simulink model "Main"  (R2020a)
settings: Solver=VariableStepAuto  StartTime=0.0  StopTime=30  RelTol=1e-3
values from neighbouring files (symbols this model uses):
  A_eq = double(A_eq)    [source_export.m]
  B_eq = double(B_eq)    [source_export.m]
  C = [1 0 0 0 0 0 0 0 0 0 0 0 ... (first row only)    [source_export.m]
  C_simulink = eye(12)    [source_export.m]
  Condition_0 = transpose([0 0 0 0 0 0 0 0 0 0 0 0])    [source_export.m]
  Condition_1 = transpose([0.2 0.2 0.2 0.2 0.2 0.2 0.2 0.2 0.2 0.2 0.2 0.2])    [source_export.m]
  D = zeros(4,4)    [source_export.m]
  D_Simulink = zeros(12,4)    [source_export.m]
  g = 9.81    [source_export.m]
  inv_G0 = inv_G_0( : , [1 , 2 ,3 ,6])    [source_export.m]
  inv_G0_LQR = inv_G_0_LQR( : , [1 , 2 ,3 ,6])    [source_export.m]
  Ixx = 8.5532e-3    (= 0.0085532)    [source_export.m]
  Iyy = 8.5532e-3    (= 0.0085532)    [source_export.m]
  Izz = 1.476e-2    (= 0.01476)    [source_export.m]
  K_q_LQR = K_LQR(:,12+1:12+4)    [source_export.m]
  K_q_LQRk = K_LQRk(:,12+1:12+4)    [source_export.m]
  Kfeedback = place(A_eq,B_eq,Poles)    [source_export.m]
  m = 1    [source_export.m]
undefined symbols (not defined in the file or in its folder): K_LQR1
libraries: simulink x1
settings Model: Creator=ali14  LastModifiedBy=ali14
settings DebuggingCC: UnconnectedInputMsg=none  UnconnectedOutputMsg=none  UnconnectedLineMsg=none  SFMachineParentedDataDiag=error
settings ModelReferenceCC: EnableRefExpFcnMdlSchedulingChecks=off
settings RTWCC: Description=Generic Real-Time Target

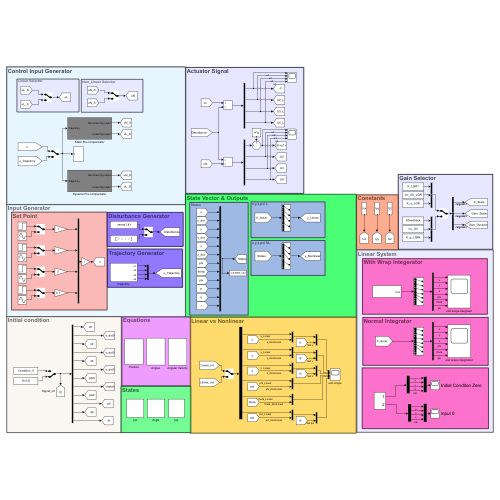
[thumbnail: Simulink's stored preview of the top-level diagram]
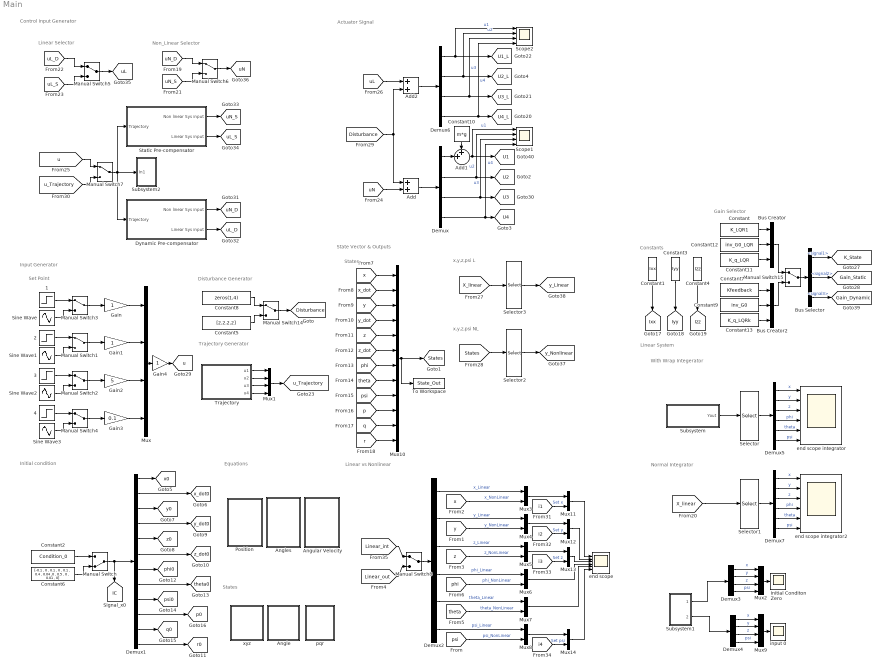
== system Main ==
  note: Gain Selector
  note: Actuator Signal
  note: States
  note: x,y,z,psi NL
  note: x,y,z,psi L
  note: Normal Integrator
  note: Trajectory Generator
  note: Linear Selector
  note: Non_Linear Selector
  note: Set Point
  note: Disturbance Generator
  note: State Vector & Outputs
  note: With Wrap Integerator
  note: Linear System
  note: Linear vs Nonlinear
  note: Constants
  note: Initial condition
  note: States
  note: Equations
  note: Input Generator
  note: Control Input Generator
  1 : Step  Time=3  SampleTime=0
  2 : Step  Time=3  SampleTime=0
  3 : Step  Time=0  SampleTime=0
  4 : Step  Time=5  SampleTime=0
  Add : Sum
  Add1 : Sum  Inputs=++|
  Add2 : Sum
  Angle : Subsystem
  Angles : Subsystem
  Angular Velocity : Subsystem
  Bus Creator : BusCreator  Inputs=3
  Bus Creator2 : BusCreator  Inputs=3
  Bus Selector : BusSelector  OutputSignals=signal1,signal2,signal3
  Constant : Constant  Value=K_LQR1
  Constant1 : Constant  Value=Ixx
  Constant10 : Constant  Value=m*g
  Constant11 : Constant  Value=K_q_LQR
  Constant12 : Constant  Value=inv_G0_LQR
  Constant13 : Constant  Value=K_q_LQRk
  Constant2 : Constant  Value=Condition_0
  Constant3 : Constant  Value=Iyy
  Constant4 : Constant  Value=Izz
  Constant5 : Constant  Value=[2,2,2,2]
  Constant6 : Constant  Value=[-0.1 , 0 , 0.1 , 0 , 0.1 , 0.4 , 0.04 ,0 , 0.5 , 0 , 0.01 , 0]
  Constant7 : Constant  Value=Kfeedback
  Constant8 : Constant  Value=zeros(1,4)
  Constant9 : Constant  Value=inv_G0
  Demux{,3..4,6} (4 alike) : Demux
  Demux1 : Demux  Outputs=12
  Demux2 : Demux  Outputs=6
  Demux5 : Demux  Outputs=6
  Demux7 : Demux  Outputs=6
  Dynamic Pre-compensator : Subsystem
  Gain : Gain
  Gain1 : Gain
  Gain2 : Gain  Gain=5
  Gain3 : Gain  Gain=0.1
  Gain4 : Gain
  Initial Conditon Zero : Scope
  Manual Switch : ManualSwitch  CurrentSetting=0
  Manual Switch{1..8,14..15} (10 alike) : ManualSwitch
  Mux{,1..2,9} (4 alike) : Mux
  Mux10 : Mux  Inputs=12
  Mux{3..8,11..14} (10 alike) : Mux  Inputs=2
  Position : Subsystem
  Scope1 : Scope  NumInputPorts=4
  Scope2 : Scope  NumInputPorts=4
  Selector : Selector  InputPortWidth=12  IndexOptions=Index vector (dialog)  Indices=[1 3 5 7 8 9]  OutputSizes=1
  Selector1 : Selector  InputPortWidth=12  IndexOptions=Index vector (dialog)  Indices=[1 3 5 7 8 9]  OutputSizes=1
  Selector2 : Selector  InputPortWidth=12  IndexOptions=Index vector (dialog)  Indices=[1 3 5 9]  OutputSizes=1
  Selector3 : Selector  InputPortWidth=12  IndexOptions=Index vector (dialog)  Indices=[1 3 5 9]  OutputSizes=1
  Sine Wave{,1..3} (4 alike) : Sin  SampleTime=0
  Static Pre-compensator : Subsystem
  Subsystem : Subsystem
  Subsystem1 : Subsystem
  Subsystem2 : Subsystem
  To Workspace : ToWorkspace  VariableName=State_Out  SampleTime=-1
  "Trajectory " : Subsystem
  end scope : Scope  NumInputPorts=6
  end scope integrator : Scope  NumInputPorts=6
  end scope integrator2 : Scope  NumInputPorts=6
  input 0 : Scope
  pqr : Subsystem
  xyz : Subsystem
  tag scope: Disturbance=global, Gain_Dynamic=global, Gain_Static=global, IC=global, Ixx=global, Iyy=global, Izz=global, K_State=global, States=global, U1=global, U1_L=global, U2=global, U2_L=global, U3=global, U3_L=global, U4=global, U4_L=global, p0=global, phi0=global, psi0=global, q0=global, r0=global, theta0=global, u=global, uL=global, uL_D=global, uL_S=global, uN=global, uN_D=global, uN_S=global, u_Trajectory=global, x0=global, x_dot0=global, y0=global, y_Linear=global, y_Nonlinear=global, y_dot0=global, z0=global, z_dot0=global
  wires:
  Demux1/1 -> [x0]
  Demux1/3 -> [y0]
  Demux1/5 -> [z0]
  Demux1/2 -> [x_dot0]
  Demux1/4 -> [y_dot0]
  Demux1/6 -> [z_dot0]
  Demux1/7 -> [phi0]
  Demux1/8 -> [theta0]
  Demux1/9 -> [psi0]
  Demux1/10 -> [p0]
  Demux1/11 -> [q0]
  Demux1/12 -> [r0]
  Constant1/1 -> [Ixx]
  Constant3/1 -> [Iyy]
  Constant4/1 -> [Izz]
  Constant6/1 -> Manual Switch/2
  Manual Switch/1 -> Demux1/1, [IC]
  Constant2/1 -> Manual Switch/1
  Demux2/1 -> Mux3/1  "x_Linear"
  [x] -> Mux3/2  "x_NonLinear"
  Demux2/2 -> Mux4/1  "y_Linear"
  Demux2/3 -> Mux5/1  "z_Linear"
  Demux2/4 -> Mux6/1  "phi_Linear"
  Demux2/5 -> Mux7/1  "theta_Linear"
  Demux2/6 -> Mux8/1  "psi_Linear"
  [y] -> Mux4/2  "y_NonLinear"
  [z] -> Mux5/2  "z_NonLinear"
  [phi] -> Mux6/2  "phi_NonLinear"
  [psi] -> Mux8/2  "psi_NonLinear"
  [theta] -> Mux7/2  "theta_NonLinear"
  Mux6/1 -> end scope/4
  Mux7/1 -> end scope/5
  Subsystem1/1(Outport) -> Demux3/1
  Demux3/1 -> Mux2/1  "x"
  Demux3/2 -> Mux2/2  "y"
  Demux3/3 -> Mux2/3  "z"
  Demux3/4 -> Mux2/4  "psi"
  Mux2/1 -> Initial Conditon Zero/1
  Demux4/2 -> Mux9/2  "y"
  Demux4/1 -> Mux9/1  "x"
  Demux4/4 -> Mux9/4  "psi"
  Demux4/3 -> Mux9/3  "z"
  Subsystem1/2(Outport1) -> Demux4/1
  Mux9/1 -> input 0/1
  Subsystem/1(Yout) -> Selector/1
  Selector/1 -> Demux5/1
  Demux5/1 -> end scope integrator/1  "x"
  Demux5/2 -> end scope integrator/2  "y"
  Demux5/3 -> end scope integrator/3  "z"
  Demux5/4 -> end scope integrator/4  "phi"
  Demux5/5 -> end scope integrator/5  "theta"
  Demux5/6 -> end scope integrator/6  "psi"
  [x] -> Mux10/1
  [x_dot] -> Mux10/2
  [y] -> Mux10/3
  [y_dot] -> Mux10/4
  [z] -> Mux10/5
  [z_dot] -> Mux10/6
  [phi] -> Mux10/7
  [theta] -> Mux10/8
  [psi] -> Mux10/9
  [p] -> Mux10/10
  [q] -> Mux10/11
  [r] -> Mux10/12
  3/1 -> Manual Switch2/1
  Gain2/1 -> Mux/3
  1/1 -> Manual Switch3/1
  Manual Switch4/1 -> Gain3/1
  Manual Switch2/1 -> Gain2/1
  Sine Wave2/1 -> Manual Switch2/2
  Gain3/1 -> Mux/4
  4/1 -> Manual Switch4/1
  Sine Wave3/1 -> Manual Switch4/2
  Sine Wave/1 -> Manual Switch3/2
  Gain/1 -> Mux/1
  Gain1/1 -> Mux/2
  Sine Wave1/1 -> Manual Switch1/2
  2/1 -> Manual Switch1/1
  Manual Switch1/1 -> Gain1/1
  Demux7/2 -> end scope integrator2/2  "y"
  Demux7/6 -> end scope integrator2/6  "psi"
  Demux7/4 -> end scope integrator2/4  "phi"
  [X_linear] -> Selector1/1
  Demux7/3 -> end scope integrator2/3  "z"
  Demux7/5 -> end scope integrator2/5  "theta"
  Selector1/1 -> Demux7/1
  Demux7/1 -> end scope integrator2/1  "x"
  Manual Switch14/1 -> [Disturbance]
  Constant8/1 -> Manual Switch14/1
  Constant5/1 -> Manual Switch14/2
  Bus Selector/1 -> [K_State]  "<signal1>"
  Demux6/1 -> Scope2/1, [U1_L]  "u1"
  Demux6/3 -> Scope2/3, [U3_L]  "u3"
  Demux6/2 -> Scope2/2, [U2_L]  "u2"
  Demux6/4 -> Scope2/4, [U4_L]  "u4"
  Demux/1 -> Add1/2
  Demux/4 -> Scope1/4, [U4]  "u4"
  Demux/3 -> Scope1/3, [U3]  "u3"
  Constant10/1 -> Add1/1
  Demux/2 -> Scope1/2, [U2]  "u2"
  Add1/1 -> Scope1/1, [U1]  "u1"
  Static Pre-compensator/2(Linear Sys input) -> [uL_S]
  Static Pre-compensator/1(Non linear Sys input) -> [uN_S]
  Dynamic Pre-compensator/2(Linear Sys input) -> [uL_D]
  Dynamic Pre-compensator/1(Non linear Sys input) -> [uN_D]
  [uN_D] -> Manual Switch6/1
  [uN_S] -> Manual Switch6/2
  [uL_S] -> Manual Switch5/2
  [uL_D] -> Manual Switch5/1
  Manual Switch6/1 -> [uN]
  Manual Switch5/1 -> [uL]
  Selector3/1 -> [y_Linear]
  Selector2/1 -> [y_Nonlinear]
  [X_linear] -> Selector3/1
  Mux10/1 -> [States], To Workspace/1
  [States] -> Selector2/1
  [uN] -> Add/2
  [Disturbance] -> Add2/2, Add/1
  Add2/1 -> Demux6/1
  Add/1 -> Demux/1
  [uL] -> Add2/1
  Constant/1 -> Bus Creator/1
  Constant12/1 -> Bus Creator/2
  Constant7/1 -> Bus Creator2/1
  Constant9/1 -> Bus Creator2/2
  Bus Creator/1 -> Manual Switch15/1
  Bus Creator2/1 -> Manual Switch15/2
  Manual Switch15/1 -> Bus Selector/1
  Bus Selector/2 -> [Gain_Static]  "<signal2>"
  Constant11/1 -> Bus Creator/3
  Constant13/1 -> Bus Creator2/3
  Bus Selector/3 -> [Gain_Dynamic]  "<signal3>"
  [u_Trajectory] -> Manual Switch7/2
  [u] -> Manual Switch7/1
  Manual Switch7/1 -> Dynamic Pre-compensator/1(Trajectory), Subsystem2/1(In1), Static Pre-compensator/1(Trajectory)
  "Trajectory "/4(u4) -> Mux1/4
  Mux1/1 -> [u_Trajectory]
  "Trajectory "/1(u1) -> Mux1/1
  "Trajectory "/2(u2) -> Mux1/2
  "Trajectory "/3(u3) -> Mux1/3
  Mux3/1 -> Mux11/1
  [i1] -> Mux11/2  "Set x"
  Mux11/1 -> end scope/1
  [i2] -> Mux12/2  "Set y"
  Mux4/1 -> Mux12/1
  Mux12/1 -> end scope/2
  [i3] -> Mux13/2  "Set z"
  Mux5/1 -> Mux13/1
  Mux13/1 -> end scope/3
  [i4] -> Mux14/2  "Set psi"
  Mux8/1 -> Mux14/1
  Mux14/1 -> end scope/6
  Manual Switch8/1 -> Demux2/1
  [Linear_out] -> Manual Switch8/2
  [Linear_int] -> Manual Switch8/1
  Manual Switch3/1 -> Gain/1
  Mux/1 -> Gain4/1
  Gain4/1 -> [u]

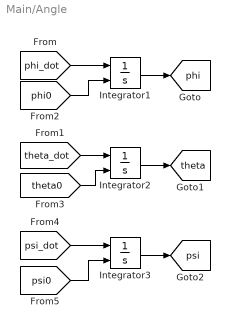
== system Main/Angle ==
  Integrator1 : Integrator  InitialConditionSource=external  WrapState=on
  Integrator2 : Integrator  InitialConditionSource=external  WrapState=on
  Integrator3 : Integrator  InitialConditionSource=external  WrapState=on
  tag scope: phi=global, psi=global, theta=global
  wires:
  Integrator2/1 -> [theta]
  [theta_dot] -> Integrator2/1
  Integrator3/1 -> [psi]
  [theta0] -> Integrator2/2
  [psi_dot] -> Integrator3/1
  [phi0] -> Integrator1/2
  Integrator1/1 -> [phi]
  [psi0] -> Integrator3/2
  [phi_dot] -> Integrator1/1

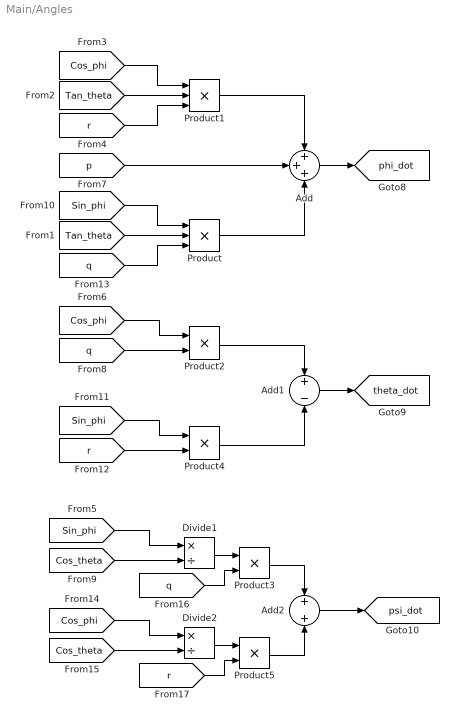
== system Main/Angles ==
  Add : Sum  Inputs=+++
  Add1 : Sum  Inputs=+-
  Add2 : Sum
  Divide1 : Product  Inputs=*/
  Divide2 : Product  Inputs=*/
  Product : Product  Inputs=3
  Product1 : Product  Inputs=3
  Product{2..5} (4 alike) : Product
  tag scope: phi_dot=global, psi_dot=global, theta_dot=global
  wires:
  [Sin_phi] -> Product/1
  [Tan_theta] -> Product/2
  [q] -> Product/3
  Product/1 -> Add/3
  [p] -> Add/2
  [Cos_phi] -> Product1/1
  [Tan_theta] -> Product1/2
  [r] -> Product1/3
  Product1/1 -> Add/1
  Add/1 -> [phi_dot]
  Add1/1 -> [theta_dot]
  [Cos_phi] -> Product2/1
  [q] -> Product2/2
  Product2/1 -> Add1/1
  Product4/1 -> Add1/2
  [Sin_phi] -> Divide1/1
  [Cos_theta] -> Divide1/2
  Divide1/1 -> Product3/1
  [r] -> Product4/2
  [Sin_phi] -> Product4/1
  Add2/1 -> [psi_dot]
  Product3/1 -> Add2/1
  [Cos_phi] -> Divide2/1
  Divide2/1 -> Product5/1
  [Cos_theta] -> Divide2/2
  Product5/1 -> Add2/2
  [q] -> Product3/2
  [r] -> Product5/2

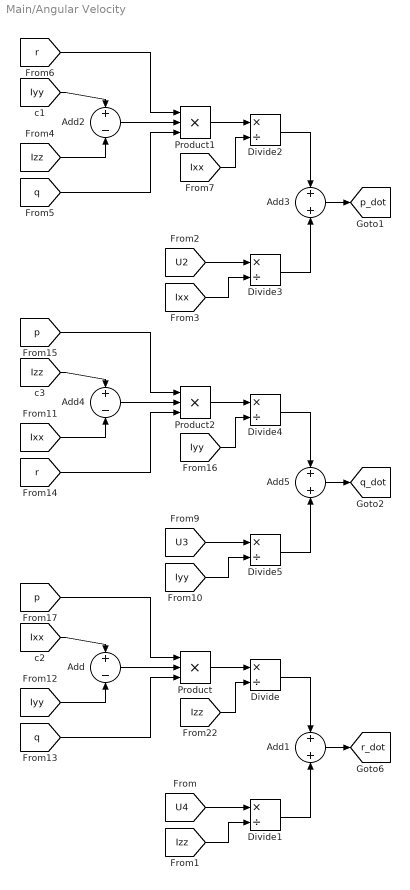
== system Main/Angular Velocity ==
  Add : Sum  Inputs=+-
  Add1 : Sum
  Add2 : Sum  Inputs=+-
  Add3 : Sum
  Add4 : Sum  Inputs=+-
  Add5 : Sum
  Divide{,1..5} (6 alike) : Product  Inputs=*/
  Product : Product  Inputs=3
  Product1 : Product  Inputs=3
  Product2 : Product  Inputs=3
  tag scope: p_dot=global, q_dot=global, r_dot=global
  wires:
  [Ixx] -> Add/1
  [Iyy] -> Add/2
  Add/1 -> Product/2
  [p] -> Product/1
  [q] -> Product/3
  Product/1 -> Divide/1
  [Izz] -> Divide/2
  Divide/1 -> Add1/1
  Add1/1 -> [r_dot]
  [U4] -> Divide1/1
  [Izz] -> Divide1/2
  Divide1/1 -> Add1/2
  [Izz] -> Add2/2
  Add2/1 -> Product1/2
  [r] -> Product1/1
  [U2] -> Divide3/1
  Add3/1 -> [p_dot]
  Divide2/1 -> Add3/1
  [Ixx] -> Divide3/2
  [q] -> Product1/3
  [Ixx] -> Divide2/2
  Product1/1 -> Divide2/1
  [Iyy] -> Add2/1
  Divide3/1 -> Add3/2
  [U3] -> Divide5/1
  [Iyy] -> Divide4/2
  Add5/1 -> [q_dot]
  [Iyy] -> Divide5/2
  Product2/1 -> Divide4/1
  [p] -> Product2/1
  Divide4/1 -> Add5/1
  [r] -> Product2/3
  Divide5/1 -> Add5/2
  [Ixx] -> Add4/2
  [Izz] -> Add4/1
  Add4/1 -> Product2/2

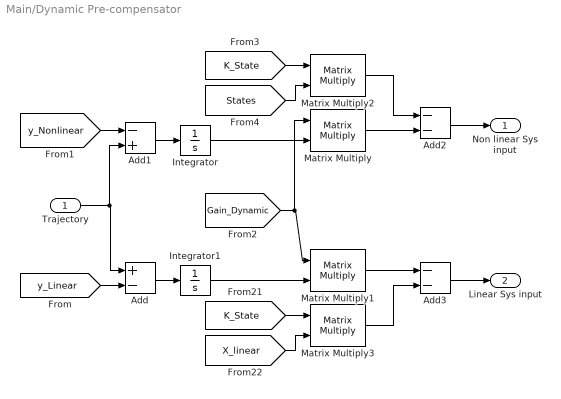
== system Main/Dynamic Pre-compensator ==
  Trajectory : Inport
  Add : Sum  Inputs=+-
  Add1 : Sum  Inputs=-+
  Add2 : Sum  Inputs=--
  Add3 : Sum  Inputs=--
  Integrator : Integrator
  Integrator1 : Integrator
  Matrix Multiply{,1..3} (4 alike) : Product  Multiplication=Matrix(*)
  Non linear Sys input : Outport
  Linear Sys input : Outport  Port=2
  wires:
  Trajectory/1 -> Add1/2, Add/1
  [y_Linear] -> Add/2
  [y_Nonlinear] -> Add1/1
  Add1/1 -> Integrator/1
  Add/1 -> Integrator1/1
  Integrator1/1 -> Matrix Multiply1/2
  [Gain_Dynamic] -> Matrix Multiply/1, Matrix Multiply1/1
  [K_State] -> Matrix Multiply3/1
  [States] -> Matrix Multiply2/2
  [K_State] -> Matrix Multiply2/1
  [X_linear] -> Matrix Multiply3/2
  Matrix Multiply/1 -> Add2/2
  Matrix Multiply2/1 -> Add2/1
  Matrix Multiply1/1 -> Add3/1
  Matrix Multiply3/1 -> Add3/2
  Add2/1 -> Non linear Sys input/1
  Add3/1 -> Linear Sys input/1
  Integrator/1 -> Matrix Multiply/2

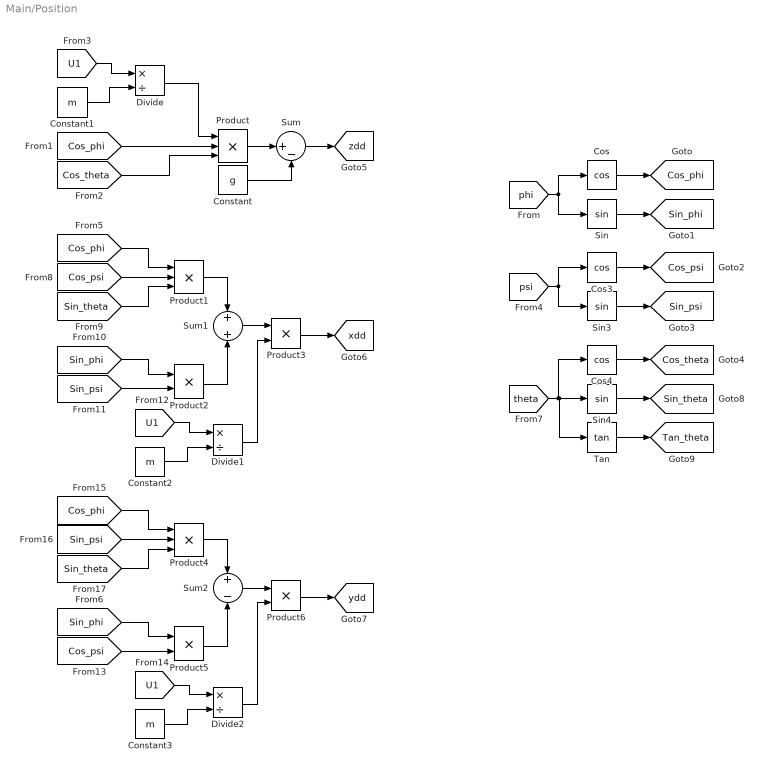
== system Main/Position ==
  Constant : Constant  Value=g
  Constant1 : Constant  Value=m
  Constant2 : Constant  Value=m
  Constant3 : Constant  Value=m
  Cos : Trigonometry  Operator=cos
  Cos3 : Trigonometry  Operator=cos
  Cos4 : Trigonometry  Operator=cos
  Divide : Product  Inputs=*/
  Divide1 : Product  Inputs=*/
  Divide2 : Product  Inputs=*/
  Product : Product  Inputs=3
  Product1 : Product  Inputs=3
  Product{2..3,5..6} (4 alike) : Product
  Product4 : Product  Inputs=3
  Sin : Trigonometry
  Sin3 : Trigonometry
  Sin4 : Trigonometry
  Sum : Sum  Inputs=|+-
  Sum1 : Sum
  Sum2 : Sum  Inputs=+-
  Tan : Trigonometry  Operator=tan
  tag scope: Cos_phi=global, Cos_psi=global, Cos_theta=global, Sin_phi=global, Sin_psi=global, Sin_theta=global, Tan_theta=global, xdd=global, ydd=global, zdd=global
  wires:
  Constant/1 -> Sum/2
  Product/1 -> Sum/1
  Sum/1 -> [zdd]
  Constant1/1 -> Divide/2
  [U1] -> Divide/1
  Divide/1 -> Product/1
  [phi] -> Cos/1, Sin/1
  Cos/1 -> [Cos_phi]
  Sin/1 -> [Sin_phi]
  Sin3/1 -> [Sin_psi]
  Cos3/1 -> [Cos_psi]
  [psi] -> Cos3/1, Sin3/1
  Sin4/1 -> [Sin_theta]
  Cos4/1 -> [Cos_theta]
  [theta] -> Cos4/1, Tan/1, Sin4/1
  [Cos_phi] -> Product/2
  [Cos_theta] -> Product/3
  [Cos_phi] -> Product1/1
  [Cos_psi] -> Product1/2
  [Sin_theta] -> Product1/3
  [Sin_psi] -> Product2/2
  [Sin_phi] -> Product2/1
  Product2/1 -> Sum1/2
  Product1/1 -> Sum1/1
  Product3/1 -> [xdd]
  Sum1/1 -> Product3/1
  Constant2/1 -> Divide1/2
  [U1] -> Divide1/1
  Divide1/1 -> Product3/2
  Product4/1 -> Sum2/1
  [Sin_theta] -> Product4/3
  Constant3/1 -> Divide2/2
  [Sin_psi] -> Product4/2
  [Cos_phi] -> Product4/1
  Product5/1 -> Sum2/2
  Divide2/1 -> Product6/2
  Sum2/1 -> Product6/1
  [Sin_phi] -> Product5/1
  [U1] -> Divide2/1
  [Cos_psi] -> Product5/2
  Product6/1 -> [ydd]
  Tan/1 -> [Tan_theta]

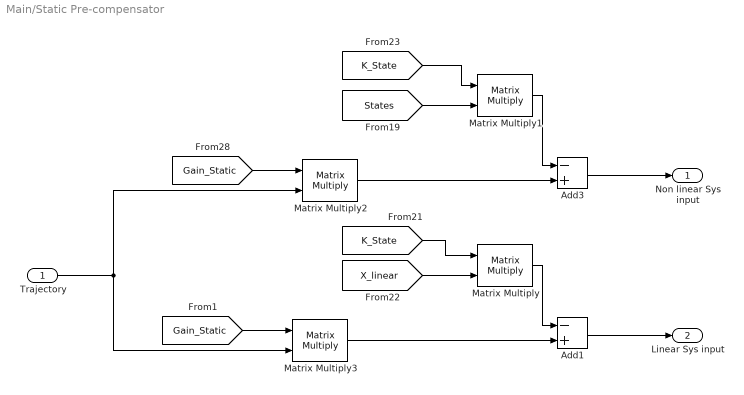
== system Main/Static Pre-compensator ==
  Trajectory : Inport
  Add1 : Sum  Inputs=-+
  Add3 : Sum  Inputs=-+
  Matrix Multiply{,1..3} (4 alike) : Product  Multiplication=Matrix(*)
  Non linear Sys input : Outport
  Linear Sys input : Outport  Port=2
  wires:
  Matrix Multiply1/1 -> Add3/1
  [States] -> Matrix Multiply1/2
  [K_State] -> Matrix Multiply1/1
  Add3/1 -> Non linear Sys input/1
  Matrix Multiply2/1 -> Add3/2
  [Gain_Static] -> Matrix Multiply2/1
  Matrix Multiply/1 -> Add1/1
  [X_linear] -> Matrix Multiply/2
  [K_State] -> Matrix Multiply/1
  Trajectory/1 -> Matrix Multiply3/2, Matrix Multiply2/2
  Matrix Multiply3/1 -> Add1/2
  [Gain_Static] -> Matrix Multiply3/1
  Add1/1 -> Linear Sys input/1

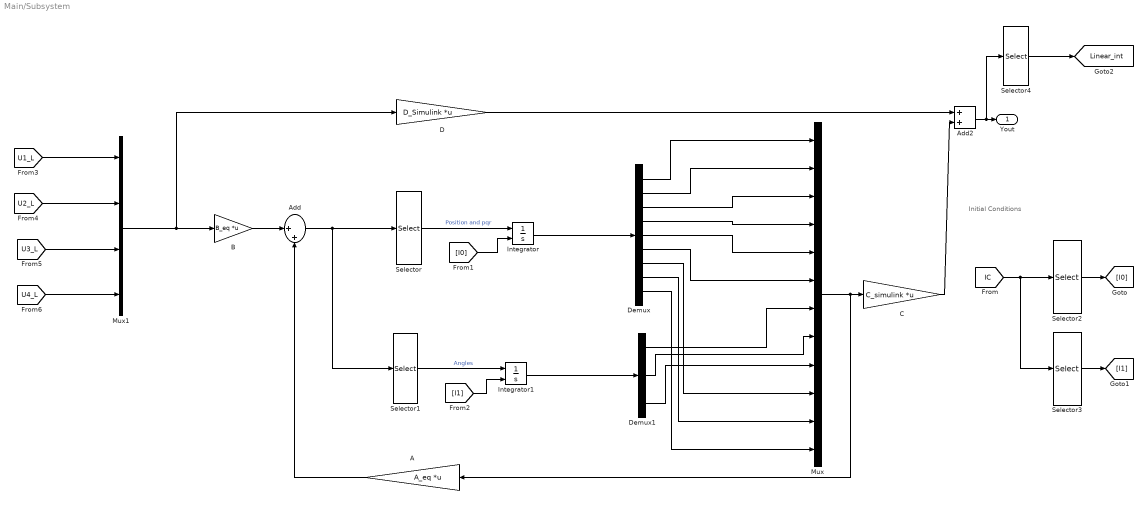
== system Main/Subsystem ==
  note: Initial Conditions
  A : Gain  Gain=A_eq  Multiplication=Matrix(K*u)
  Add : Sum  Inputs=|++
  Add2 : Sum
  B : Gain  Gain=B_eq  Multiplication=Matrix(K*u)
  C : Gain  Gain=C_simulink  Multiplication=Matrix(K*u)
  D : Gain  Gain=D_Simulink  Multiplication=Matrix(K*u)
  Demux : Demux  Outputs=9
  Demux1 : Demux  Outputs=3
  Integrator : Integrator  InitialConditionSource=external
  Integrator1 : Integrator  InitialConditionSource=external  WrapState=on
  Mux : Mux  Inputs=12
  Mux1 : Mux
  Selector : Selector  InputPortWidth=12  IndexOptions=Index vector (dialog)  Indices=[1 2 3 4 5 6 10 11 12]  OutputSizes=1
  Selector1 : Selector  InputPortWidth=12  IndexOptions=Index vector (dialog)  Indices=[7 8 9]  OutputSizes=1
  Selector2 : Selector  InputPortWidth=12  IndexOptions=Index vector (dialog)  Indices=[1 2 3 4 5 6 10 11 12]  OutputSizes=1
  Selector3 : Selector  InputPortWidth=12  IndexOptions=Index vector (dialog)  Indices=[7 8 9]  OutputSizes=1
  Selector4 : Selector  InputPortWidth=12  IndexOptions=Index vector (dialog)  Indices=[1 3 5 7 8 9]  OutputSizes=1
  Yout : Outport
  tag scope: Linear_int=global
  wires:
  B/1 -> Add/1
  A/1 -> Add/2
  Add/1 -> Selector1/1, Selector/1
  Selector/1 -> Integrator/1  "Position and pqr"
  Selector1/1 -> Integrator1/1  "Angles"
  [IC] -> Selector3/1, Selector2/1
  Selector3/1 -> [I1]
  Selector2/1 -> [I0]
  [I1] -> Integrator1/2
  [I0] -> Integrator/2
  Integrator1/1 -> Demux1/1
  Integrator/1 -> Demux/1
  Demux/1 -> Mux/1
  Demux/2 -> Mux/2
  Demux/3 -> Mux/3
  Demux/4 -> Mux/4
  Demux/5 -> Mux/5
  Demux/6 -> Mux/6
  Demux1/1 -> Mux/7
  Demux1/2 -> Mux/8
  Demux1/3 -> Mux/9
  Demux/7 -> Mux/10
  Demux/8 -> Mux/11
  Demux/9 -> Mux/12
  D/1 -> Add2/1
  C/1 -> Add2/2
  Mux1/1 -> D/1, B/1
  [U2_L] -> Mux1/2
  [U3_L] -> Mux1/3
  [U4_L] -> Mux1/4
  Add2/1 -> Selector4/1, Yout/1
  Mux/1 -> A/1, C/1
  [U1_L] -> Mux1/1
  Selector4/1 -> [Linear_int]

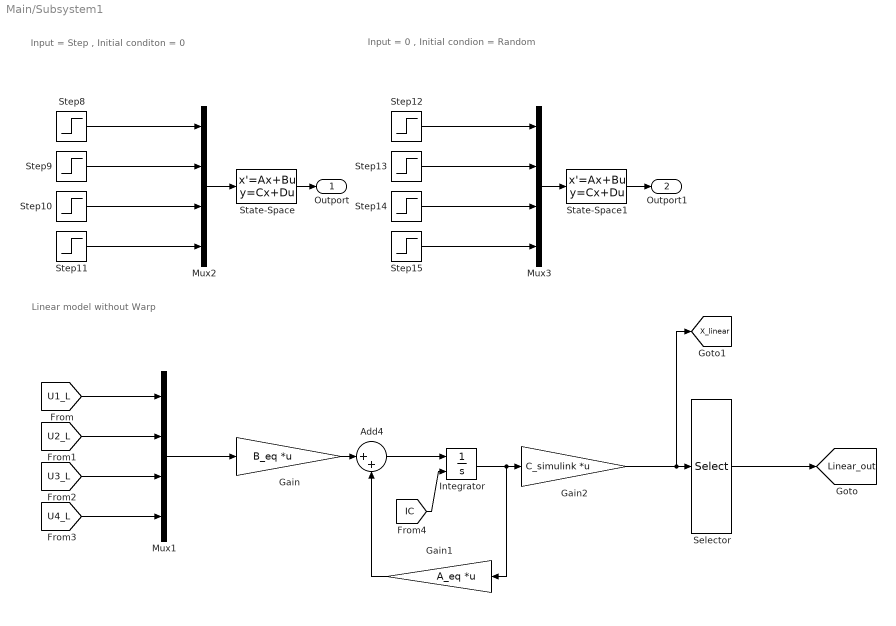
== system Main/Subsystem1 ==
  note: Linear model without Warp
  note: Input = Step , Initial conditon = 0
  note: Input = 0 , Initial condion = Random
  Add4 : Sum  Inputs=|++
  Gain : Gain  Gain=B_eq  Multiplication=Matrix(K*u)
  Gain1 : Gain  Gain=A_eq  Multiplication=Matrix(K*u)
  Gain2 : Gain  Gain=C_simulink  Multiplication=Matrix(K*u)
  Integrator : Integrator  InitialConditionSource=external
  Mux1 : Mux
  Mux2 : Mux
  Mux3 : Mux
  Selector : Selector  InputPortWidth=12  IndexOptions=Index vector (dialog)  Indices=[1 3 5 7 8 9]  OutputSizes=1
  State-Space : StateSpace  A=A_eq  B=B_eq  C=C  D=D  InitialCondition=Condition_0
  State-Space1 : StateSpace  A=A_eq  B=B_eq  C=C  D=D  InitialCondition=Condition_1
  Step{8..11} (4 alike) : Step  Time=0  SampleTime=0
  Step{12..15} (4 alike) : Step  Time=0  After=0  SampleTime=0
  Outport : Outport
  Outport1 : Outport  Port=2
  tag scope: Linear_out=global, X_linear=global
  wires:
  State-Space1/1 -> Outport1/1
  Step15/1 -> Mux3/4
  Step11/1 -> Mux2/4
  Step9/1 -> Mux2/2
  Mux3/1 -> State-Space1/1
  Step10/1 -> Mux2/3
  State-Space/1 -> Outport/1
  Step13/1 -> Mux3/2
  Mux2/1 -> State-Space/1
  Step14/1 -> Mux3/3
  [U2_L] -> Mux1/2
  [U3_L] -> Mux1/3
  [U4_L] -> Mux1/4
  Step12/1 -> Mux3/1
  [U1_L] -> Mux1/1
  Selector/1 -> [Linear_out]
  [IC] -> Integrator/2
  Integrator/1 -> Gain1/1, Gain2/1
  Gain1/1 -> Add4/2
  Mux1/1 -> Gain/1
  Gain/1 -> Add4/1
  Gain2/1 -> [X_linear], Selector/1
  Add4/1 -> Integrator/1
  Step8/1 -> Mux2/1

== system Main/Subsystem2 ==
  In1 : Inport
  Demux8 : Demux
  tag scope: i1=global, i2=global, i3=global, i4=global
  wires:
  In1/1 -> Demux8/1
  Demux8/1 -> [i1]
  Demux8/2 -> [i2]
  Demux8/3 -> [i3]
  Demux8/4 -> [i4]

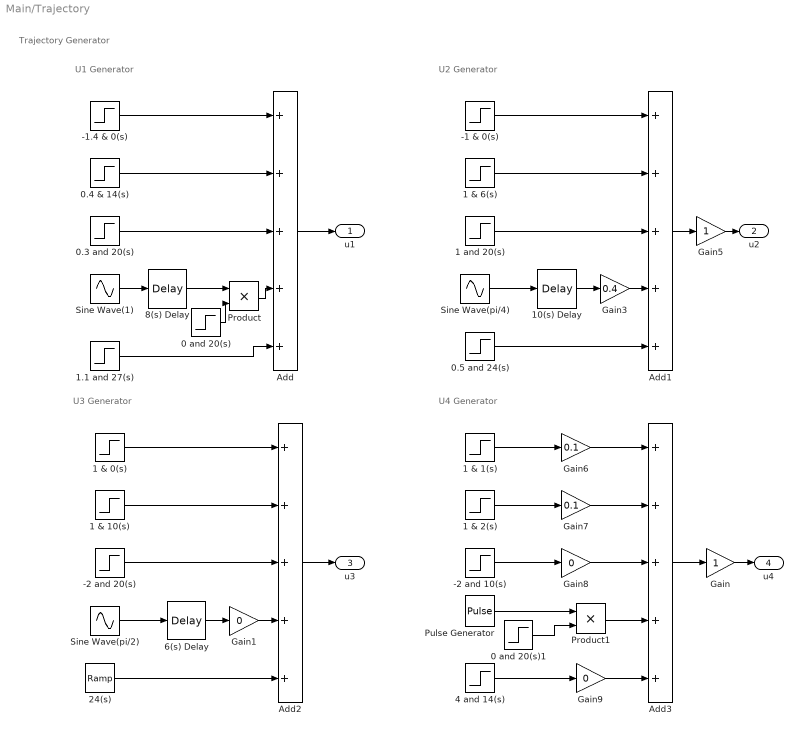
== system Main/Trajectory  ==
  note: U4 Generator
  note: U3 Generator
  note: U2 Generator
  note: U1 Generator
  note: Trajectory Generator
  -1 & 0(s) : Step  Time=0  After=-1  SampleTime=0
  -1.4 & 0(s) : Step  Time=0  After=-1.4  SampleTime=0
  -2 and 10(s) : Step  Time=10  After=-2  SampleTime=0
  -2 and 20(s) : Step  Time=20  After=-2  SampleTime=0
  0 and 20(s) : Step  Time=20  Before=1  After=0  SampleTime=0
  0 and 20(s)1 : Step  Time=20  Before=1  After=0  SampleTime=0
  0.3 and 20(s) : Step  Time=20  After=0.3  SampleTime=0
  0.4 & 14(s) : Step  Time=14  After=0.4  SampleTime=0
  0.5 and 24(s) : Step  Time=24  After=0.5  SampleTime=0
  1 & 0(s) : Step  Time=0  After=-1  SampleTime=0
  1 & 1(s) : Step  SampleTime=0
  1 & 10(s) : Step  Time=10  After=2  SampleTime=0
  1 & 2(s) : Step  Time=2  After=-1  SampleTime=0
  1 & 6(s) : Step  Time=6  SampleTime=0
  1 and 20(s) : Step  Time=20  SampleTime=0
  1.1 and 27(s) : Step  Time=27  After=1.1  SampleTime=0
  10(s) Delay : TransportDelay  DelayTime=10  BufferSize=2048
  24(s) : simulink/Sources/Ramp  slope=1  start=24  InitialOutput=0
  4 and 14(s) : Step  Time=12  After=4  SampleTime=0
  6(s) Delay : TransportDelay  DelayTime=6
  8(s) Delay : TransportDelay  DelayTime=8  BufferSize=2048
  Add{,1..3} (4 alike) : Sum  Inputs=+++++
  Gain : Gain
  Gain1 : Gain  Gain=0
  Gain3 : Gain  Gain=0.4
  Gain5 : Gain
  Gain6 : Gain  Gain=0.1
  Gain7 : Gain  Gain=0.1
  Gain8 : Gain  Gain=0
  Gain9 : Gain  Gain=0
  Product : Product
  Product1 : Product
  Pulse Generator : DiscretePulseGenerator  PulseType=Time based  Period=5  PulseWidth=30  PhaseDelay=5
  Sine Wave(1) : Sin  Amplitude=0.4  SampleTime=0
  Sine Wave(pi/2) : Sin  Amplitude=0.4  Frequency=pi/2  SampleTime=0
  Sine Wave(pi/4) : Sin  Frequency=pi/4  SampleTime=0
  u1 : Outport
  u2 : Outport  Port=2
  u3 : Outport  Port=3
  u4 : Outport  Port=4
  wires:
  Add/1 -> u1/1
  Sine Wave(1)/1 -> 8(s) Delay/1
  -1.4 & 0(s)/1 -> Add/1
  0.3 and 20(s)/1 -> Add/3
  8(s) Delay/1 -> Product/1
  0.4 & 14(s)/1 -> Add/2
  1.1 and 27(s)/1 -> Add/5
  Sine Wave(pi/4)/1 -> 10(s) Delay/1
  0.5 and 24(s)/1 -> Add1/5
  10(s) Delay/1 -> Gain3/1
  1 & 6(s)/1 -> Add1/2
  -1 & 0(s)/1 -> Add1/1
  1 and 20(s)/1 -> Add1/3
  Add2/1 -> u3/1
  -2 and 20(s)/1 -> Add2/3
  24(s)/1 -> Add2/5
  Sine Wave(pi/2)/1 -> 6(s) Delay/1
  1 & 10(s)/1 -> Add2/2
  1 & 0(s)/1 -> Add2/1
  6(s) Delay/1 -> Gain1/1
  Add3/1 -> Gain/1
  4 and 14(s)/1 -> Gain9/1
  1 & 1(s)/1 -> Gain6/1
  -2 and 10(s)/1 -> Gain8/1
  1 & 2(s)/1 -> Gain7/1
  Gain/1 -> u4/1
  Gain1/1 -> Add2/4
  Gain3/1 -> Add1/4
  Product/1 -> Add/4
  Add1/1 -> Gain5/1
  Gain5/1 -> u2/1
  Gain6/1 -> Add3/1
  Gain7/1 -> Add3/2
  Gain8/1 -> Add3/3
  Gain9/1 -> Add3/5
  0 and 20(s)/1 -> Product/2
  Product1/1 -> Add3/4
  Pulse Generator/1 -> Product1/1
  0 and 20(s)1/1 -> Product1/2

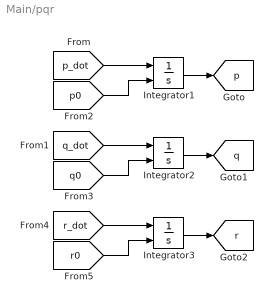
== system Main/pqr ==
  Integrator1 : Integrator  InitialConditionSource=external
  Integrator2 : Integrator  InitialConditionSource=external
  Integrator3 : Integrator  InitialConditionSource=external
  tag scope: p=global, q=global, r=global
  wires:
  [q0] -> Integrator2/2
  [q_dot] -> Integrator2/1
  Integrator2/1 -> [q]
  Integrator1/1 -> [p]
  [p_dot] -> Integrator1/1
  [p0] -> Integrator1/2
  [r_dot] -> Integrator3/1
  [r0] -> Integrator3/2
  Integrator3/1 -> [r]

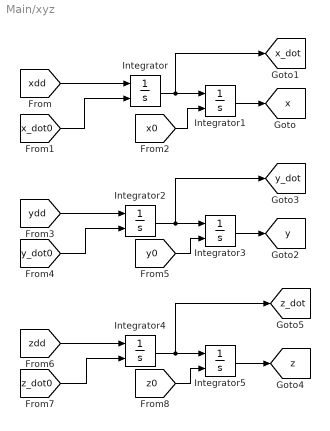
== system Main/xyz ==
  Integrator{,1..5} (6 alike) : Integrator  InitialConditionSource=external
  tag scope: x=global, x_dot=global, y=global, y_dot=global, z=global, z_dot=global
  wires:
  Integrator3/1 -> [y]
  [z0] -> Integrator5/2
  [x0] -> Integrator1/2
  Integrator2/1 -> [y_dot], Integrator3/1
  [y0] -> Integrator3/2
  Integrator/1 -> Integrator1/1, [x_dot]
  Integrator1/1 -> [x]
  Integrator4/1 -> [z_dot], Integrator5/1
  Integrator5/1 -> [z]
  [z_dot0] -> Integrator4/2
  [zdd] -> Integrator4/1
  [y_dot0] -> Integrator2/2
  [ydd] -> Integrator2/1
  [x_dot0] -> Integrator/2
  [xdd] -> Integrator/1
